simulink model "Project1_Assignment"  (R2014a)
settings: Solver=ode3  StartTime=0.0  StopTime=30  FixedStep=0.01  RelTol=1e-3
libraries: simulink x1
settings Model: Creator=dzr3qn  LastModifiedBy=dzr3qn

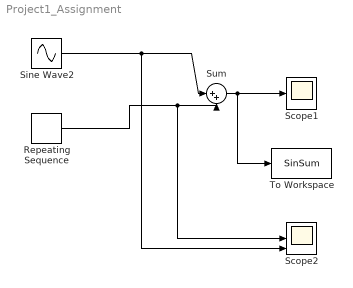
== system Project1_Assignment ==
  Repeating Sequence : simulink/Sources/Repeating Sequence  rep_seq_t=[0 1]  rep_seq_y=[0 4]
  Scope1 : Scope
      settings: TimeRange=30
  Scope2 : Scope  NumInputPorts=3
      settings: YMin=-5~-5~-5  YMax=5~5~5  SaveName=ScopeData2
  Sine Wave2 : Sin  Amplitude=5  SampleTime=0
  Sum : Sum  Inputs=|++
  To Workspace : ToWorkspace  VariableName=SinSum  SaveFormat=Timeseries  SampleTime=-1
  wires:
  Sum/1 -> To Workspace/1, Scope1/1
  Sine Wave2/1 -> Scope2/3, Sum/1
  Repeating Sequence/1 -> Scope2/2, Sum/2
